simulink model "myModel1"  (R2020a)
settings: Solver=VariableStepAuto  StartTime=0.0  StopTime=0.5  RelTol=1e-3
settings Model: Creator=assetmalik  LastModifiedBy=assetmalik

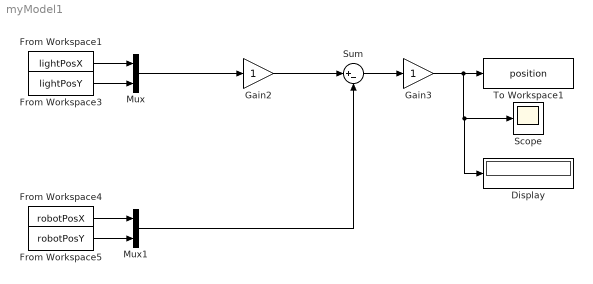
== system myModel1 ==
  Display : Display
  From Workspace1 : FromWorkspace  VariableName=lightPosX
  From Workspace3 : FromWorkspace  VariableName=lightPosY
  From Workspace4 : FromWorkspace  VariableName=robotPosX
  From Workspace5 : FromWorkspace  VariableName=robotPosY
  Gain2 : Gain
  Gain3 : Gain
  Mux : Mux  Inputs=2
  Mux1 : Mux  Inputs=2
  Scope : Scope
  Sum : Sum  Inputs=|+-
  To Workspace1 : ToWorkspace  VariableName=position  SaveFormat=Timeseries  SampleTime=-1
  wires:
  Gain2/1 -> Sum/1
  Gain3/1 -> Display/1, Scope/1, To Workspace1/1
  Sum/1 -> Gain3/1
  Mux/1 -> Gain2/1
  From Workspace1/1 -> Mux/1
  From Workspace3/1 -> Mux/2
  From Workspace5/1 -> Mux1/2
  From Workspace4/1 -> Mux1/1
  Mux1/1 -> Sum/2
